simulink model "M313"  (R2021b)
settings: Solver=VariableStepAuto  StartTime=0.0  StopTime=10.0  RelTol=1e-3
settings Model: Creator=abdul  LastModifiedBy=abdul

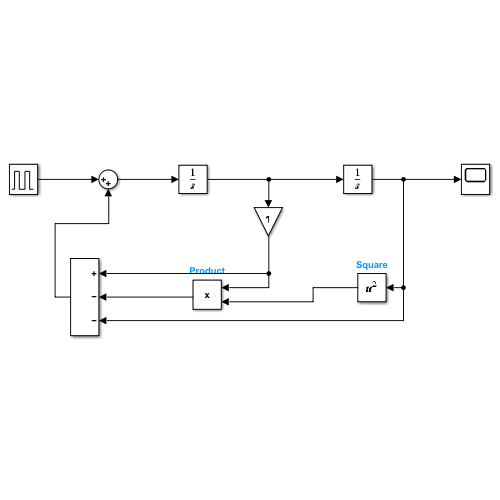
[thumbnail: Simulink's stored preview of the top-level diagram]
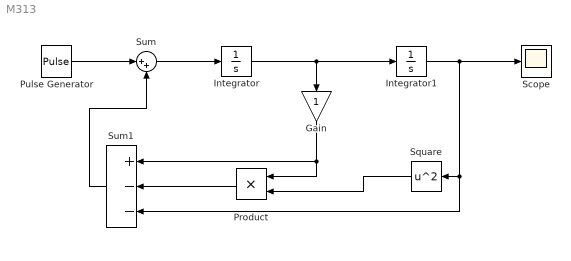
== system M313 ==
  Gain : Gain
  Integrator : Integrator
  Integrator1 : Integrator
  Product : Product
  Pulse Generator : DiscretePulseGenerator  PulseType=Time based  Period=10  PulseWidth=5
  Scope : Scope
  Square : Math  Operator=square  SaturateOnIntegerOverflow=on
  Sum : Sum  Inputs=|++
  Sum1 : Sum  Inputs=+--
  wires:
  Integrator/1 -> Gain/1, Integrator1/1
  Integrator1/1 -> Sum1/3, Square/1, Scope/1
  Gain/1 -> Sum1/1, Product/1
  Square/1 -> Product/2
  Product/1 -> Sum1/2
  Sum1/1 -> Sum/2
  Pulse Generator/1 -> Sum/1
  Sum/1 -> Integrator/1
